simulink model "gm_dsp_proj_v3_2024_n"  (R2025b)
settings: Solver=FixedStepDiscrete  StartTime=0.0  StopTime=1e-4  FixedStep=1.66666666666667e-08  RelTol=1e-3
undefined symbols (not defined in the file or in its folder): b_1, b_2, b_3, dspblkCoreblockFVToolHelper, gcbh
libraries: hdlsllib x11, simulink x4
settings Model: Creator=UTSAB KARAN  LastModifiedBy=souma
settings SolverCC: AutoInsertRateTranBlk=on
settings OptimizationCC: BlockReduction=off  ConditionallyExecuteInputs=off
settings DebuggingCC: InheritedTsInSrcMsg=none  SingleTaskRateTransMsg=error

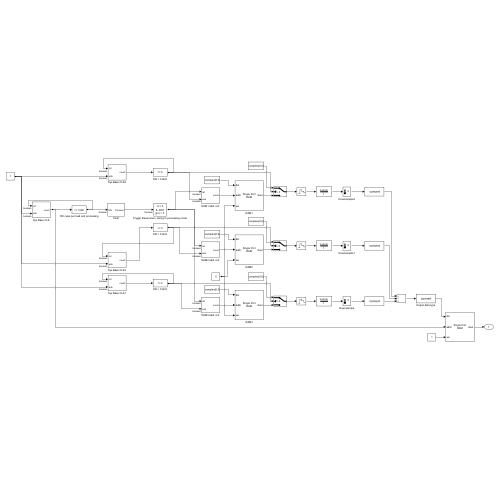
[thumbnail: Simulink's stored preview of the top-level diagram]
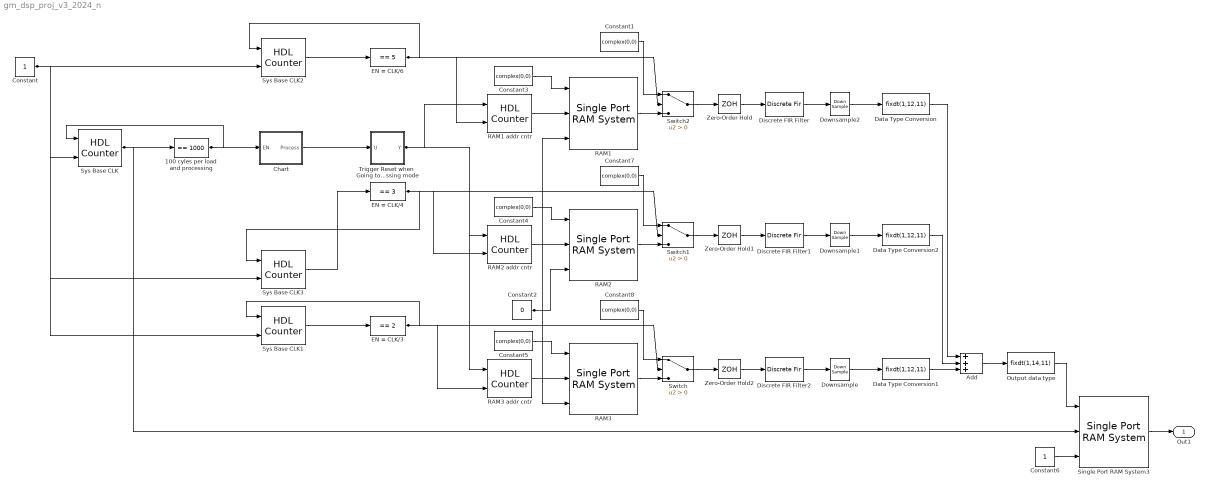
== system gm_dsp_proj_v3_2024_n ==
  100 cyles per load and processing : simulink/Logic and Bit Operations/Compare To Constant  relop===  const=1000  OutDataTypeStr=boolean
  Add : Sum  Inputs=+++  OutDataTypeStr=fixdt(1, 16, 11)
  Chart : Subsystem
  Constant : Constant  OutDataTypeStr=boolean
  Constant1 : Constant  Value=complex(0,0)  VectorParams1D=off  OutDataTypeStr=fixdt(1,8,6)  SampleTime=-1  LockScale=on
  Constant2 : Constant  Value=0  OutDataTypeStr=boolean
  Constant3 : Constant  Value=complex(0,0)  OutDataTypeStr=fixdt(1,8,6)
  Constant4 : Constant  Value=complex(0,0)  OutDataTypeStr=fixdt(1,10,8)
  Constant5 : Constant  Value=complex(0,0)  OutDataTypeStr=fixdt(1,12,10)
  Constant6 : Constant  OutDataTypeStr=boolean
  Constant7 : Constant  Value=complex(0,0)  VectorParams1D=off  OutDataTypeStr=fixdt(1,10,8)  SampleTime=-1  LockScale=on
  Constant8 : Constant  Value=complex(0,0)  VectorParams1D=off  OutDataTypeStr=fixdt(1,12,10)  SampleTime=-1  LockScale=on
  Data Type Conversion : DataTypeConversion  OutDataTypeStr=fixdt(1,12,11)  RndMeth=Floor
  Data Type Conversion1 : DataTypeConversion  OutDataTypeStr=fixdt(1,12,11)  RndMeth=Floor
  Data Type Conversion2 : DataTypeConversion  OutDataTypeStr=fixdt(1,12,11)  RndMeth=Floor
  Discrete FIR Filter : DiscreteFir  LoadFcn=dspblkCoreblockFVToolHelper(gcbh,'load');  FilterStructure=Direct form symmetric  Coefficients=b_1  CoefDataTypeStr=fixdt(1,25,24)  OutDataTypeStr=fixdt(1, 64, 30)
      settings: CopyFcn=dspblkCoreblockFVToolHelper(gcbh,'copy');  DeleteFcn=dspblkCoreblockFVToolHelper(gcbh,'close');  ModelCloseFcn=dspblkCoreblockFVToolHelper(gcbh,'close');  PreSaveFcn=dspblkCoreblockFVToolHelper(gcbh,'presave');  PostSaveFcn=dspblkCoreblockFVToolHelper(gcbh,'postsave');  CloseFcn=dspblkCoreblockFVToolHelper(gcbh,'close');
  Discrete FIR Filter1 : DiscreteFir  LoadFcn=dspblkCoreblockFVToolHelper(gcbh,'load');  FilterStructure=Direct form symmetric  Coefficients=b_2  CoefDataTypeStr=fixdt(1,25,24)  OutDataTypeStr=fixdt(1, 64, 32)
      settings: CopyFcn=dspblkCoreblockFVToolHelper(gcbh,'copy');  DeleteFcn=dspblkCoreblockFVToolHelper(gcbh,'close');  ModelCloseFcn=dspblkCoreblockFVToolHelper(gcbh,'close');  PreSaveFcn=dspblkCoreblockFVToolHelper(gcbh,'presave');  PostSaveFcn=dspblkCoreblockFVToolHelper(gcbh,'postsave');  CloseFcn=dspblkCoreblockFVToolHelper(gcbh,'close');
  Discrete FIR Filter2 : DiscreteFir  LoadFcn=dspblkCoreblockFVToolHelper(gcbh,'load');  FilterStructure=Direct form symmetric  Coefficients=b_3  CoefDataTypeStr=fixdt(1,25,24)  OutDataTypeStr=fixdt(1, 64, 34)
      settings: CopyFcn=dspblkCoreblockFVToolHelper(gcbh,'copy');  DeleteFcn=dspblkCoreblockFVToolHelper(gcbh,'close');  ModelCloseFcn=dspblkCoreblockFVToolHelper(gcbh,'close');  PreSaveFcn=dspblkCoreblockFVToolHelper(gcbh,'presave');  PostSaveFcn=dspblkCoreblockFVToolHelper(gcbh,'postsave');  CloseFcn=dspblkCoreblockFVToolHelper(gcbh,'close');
  Downsample : DownSample  N=5  RateOptions=Allow multirate processing
  Downsample1 : DownSample  N=5  RateOptions=Allow multirate processing
  Downsample2 : DownSample  N=5  RateOptions=Allow multirate processing
  EN = CLK/3 : simulink/Logic and Bit Operations/Compare To Constant  relop===  const=2  OutDataTypeStr=boolean
  EN = CLK/4 : simulink/Logic and Bit Operations/Compare To Constant  relop===  const=3  OutDataTypeStr=boolean
  EN = CLK/6 : simulink/Logic and Bit Operations/Compare To Constant  relop===  const=5  OutDataTypeStr=boolean
  Output data type : DataTypeConversion  OutDataTypeStr=fixdt(1,14,11)  SaturateOnIntegerOverflow=off  RndMeth=Floor  LockScale=on
  RAM1 : hdlsllib/HDL RAMs/Single Port RAM System  RAMType=Single port  AsyncRead=off  WriteOutputValue=New data  RAMInitialValue=ram1_init_data  allowBusInputs=off  WritesHaveOutput=on  NumReads=0  NumWrites=1  SimulateUsing=Code generation  ModelRAMDelay=on  VectorAccess=Parallel
  RAM1 addr cntr : hdlsllib/Sources/HDL Counter  CountType=Count limited  CountInit=0  CountStep=1  CountMax=3000  CountFromType=Initial value  CountFrom=0  CountResetPort=on  CountLoadPort=off  CountEnbPort=on  CountDirPort=off  CountHitOutputPort=off  CountDataType=Unsigned  CountWordLen=12  CountFracLen=0  CountSampTime=1
  RAM2 : hdlsllib/HDL RAMs/Single Port RAM System  RAMType=Single port  AsyncRead=off  WriteOutputValue=New data  RAMInitialValue=ram2_init_data  allowBusInputs=off  WritesHaveOutput=on  NumReads=0  NumWrites=1  SimulateUsing=Code generation  ModelRAMDelay=on  VectorAccess=Parallel
  RAM2 addr cntr : hdlsllib/Sources/HDL Counter  CountType=Count limited  CountInit=0  CountStep=1  CountMax=3000  CountFromType=Initial value  CountFrom=0  CountResetPort=on  CountLoadPort=off  CountEnbPort=on  CountDirPort=off  CountHitOutputPort=off  CountDataType=Unsigned  CountWordLen=12  CountFracLen=0  CountSampTime=1
  RAM3 : hdlsllib/HDL RAMs/Single Port RAM System  RAMType=Single port  AsyncRead=off  WriteOutputValue=New data  RAMInitialValue=ram3_init_data  allowBusInputs=off  WritesHaveOutput=on  NumReads=0  NumWrites=1  SimulateUsing=Code generation  ModelRAMDelay=on  VectorAccess=Parallel
  RAM3 addr cntr : hdlsllib/Sources/HDL Counter  CountType=Count limited  CountInit=0  CountStep=1  CountMax=3000  CountFromType=Initial value  CountFrom=0  CountResetPort=on  CountLoadPort=off  CountEnbPort=on  CountDirPort=off  CountHitOutputPort=off  CountDataType=Unsigned  CountWordLen=12  CountFracLen=0  CountSampTime=1
  Single Port RAM System3 : hdlsllib/HDL RAMs/Single Port RAM System  RAMType=Single port  AsyncRead=off  WriteOutputValue=New data  RAMInitialValue=0  allowBusInputs=off  WritesHaveOutput=on  NumReads=0  NumWrites=1  SimulateUsing=Code generation  ModelRAMDelay=on  VectorAccess=Parallel
  Switch : Switch  Criteria=u2 > Threshold  OutDataTypeStr=fixdt(1, 12, 10)  SaturateOnIntegerOverflow=off  InputSameDT=off
  Switch1 : Switch  Criteria=u2 > Threshold  OutDataTypeStr=fixdt(1, 10, 8)  SaturateOnIntegerOverflow=off  InputSameDT=off
  Switch2 : Switch  Criteria=u2 > Threshold  OutDataTypeStr=fixdt(1, 8, 6)  SaturateOnIntegerOverflow=off  InputSameDT=off
  Sys Base CLK : hdlsllib/Sources/HDL Counter  CountType=Count limited  CountInit=0  CountStep=1  CountMax=1000  CountFromType=Initial value  CountFrom=0  CountResetPort=on  CountLoadPort=off  CountEnbPort=on  CountDirPort=off  CountHitOutputPort=off  CountDataType=Unsigned  CountWordLen=12  CountFracLen=0  CountSampTime=1
  Sys Base CLK1 : hdlsllib/Sources/HDL Counter  CountType=Count limited  CountInit=0  CountStep=1  CountMax=2  CountFromType=Initial value  CountFrom=0  CountResetPort=on  CountLoadPort=off  CountEnbPort=on  CountDirPort=off  CountHitOutputPort=off  CountDataType=Unsigned  CountWordLen=12  CountFracLen=0  CountSampTime=1
  Sys Base CLK2 : hdlsllib/Sources/HDL Counter  CountType=Count limited  CountInit=0  CountStep=1  CountMax=5  CountFromType=Initial value  CountFrom=0  CountResetPort=on  CountLoadPort=off  CountEnbPort=on  CountDirPort=off  CountHitOutputPort=off  CountDataType=Unsigned  CountWordLen=12  CountFracLen=0  CountSampTime=1
  Sys Base CLK3 : hdlsllib/Sources/HDL Counter  CountType=Count limited  CountInit=0  CountStep=1  CountMax=3  CountFromType=Initial value  CountFrom=0  CountResetPort=on  CountLoadPort=off  CountEnbPort=on  CountDirPort=off  CountHitOutputPort=off  CountDataType=Unsigned  CountWordLen=12  CountFracLen=0  CountSampTime=1
  Trigger Reset when  Going to processing mode : Subsystem  mask(Detect Rise Positive){vinit=double(0), InputProcessing=Elements as channels (sample based), OutDataTypeStr=boolean}
      mask prompts: vinit "Simulink:masks:InitialCondition_MP"; InputProcessing "Simulink:masks:InputProcessing_MP"; OutDataTypeStr "Simulink:masks:OutputDataType_MP"
      mask help: Simulink:masks:DetectRisePositive_MD
      mask init:
      | InputProcessing = 'Elements as channels (sample based)';
      | OutDataTypeStr = 'boolean';
      | vinit = double(0);
      mask TypeOptions InputProcessing: Simulink:masks:ColumnsAsChannelsFrameBased | Simulink:masks:ElementsAsChannelsSampleBased
      mask TypeOptions OutDataTypeStr: Simulink:masks:uint8 | Simulink:masks:boolean
      mask Display: fprintf('U > 0\n&  NOT\nU/z > 0')
  Zero-Order Hold : ZeroOrderHold  SampleTime=1/60e6
  Zero-Order Hold1 : ZeroOrderHold  SampleTime=1/60e6
  Zero-Order Hold2 : ZeroOrderHold  SampleTime=1/60e6
  Out1 : Outport  SampleTime=8.33333333333333e-08
  wires:
  Constant/1 -> Sys Base CLK3/2, Sys Base CLK1/2, Sys Base CLK2/2, Sys Base CLK/2
  100 cyles per load and processing/1 -> Sys Base CLK/1, Chart/1(EN)
  Sys Base CLK/1 -> 100 cyles per load and processing/1, Single Port RAM System3/2
  Sys Base CLK2/1 -> EN = CLK/6/1
  Sys Base CLK1/1 -> EN = CLK/3/1
  Sys Base CLK3/1 -> EN = CLK/4/1
  Switch2/1 -> Zero-Order Hold/1
  Chart/1(Process) -> Trigger Reset when  Going to processing mode/1(U)
  Constant7/1 -> Switch1/1
  EN = CLK/6/1 -> Sys Base CLK2/1, Switch2/2, RAM1 addr cntr/2
  Trigger Reset when  Going to processing mode/1(Y) -> RAM1 addr cntr/1, RAM3 addr cntr/1, RAM2 addr cntr/1
  EN = CLK/4/1 -> Sys Base CLK3/1, Switch1/2, RAM2 addr cntr/2
  RAM3/1 -> Switch/3
  Constant8/1 -> Switch/1
  RAM3 addr cntr/1 -> RAM3/2
  EN = CLK/3/1 -> Sys Base CLK1/1, Switch/2, RAM3 addr cntr/2
  Constant3/1 -> RAM1/1
  RAM1 addr cntr/1 -> RAM1/2
  Constant4/1 -> RAM2/1
  Output data type/1 -> Single Port RAM System3/1
  RAM2 addr cntr/1 -> RAM2/2
  Downsample2/1 -> Data Type Conversion/1
  Constant2/1 -> RAM1/3, RAM3/3, RAM2/3
  Discrete FIR Filter2/1 -> Downsample/1
  Constant5/1 -> RAM3/1
  Constant1/1 -> Switch2/1
  RAM1/1 -> Switch2/3
  RAM2/1 -> Switch1/3
  Data Type Conversion1/1 -> Add/3
  Switch1/1 -> Zero-Order Hold1/1
  Switch/1 -> Zero-Order Hold2/1
  Zero-Order Hold/1 -> Discrete FIR Filter/1
  Zero-Order Hold1/1 -> Discrete FIR Filter1/1
  Zero-Order Hold2/1 -> Discrete FIR Filter2/1
  Discrete FIR Filter/1 -> Downsample2/1
  Discrete FIR Filter1/1 -> Downsample1/1
  Downsample1/1 -> Data Type Conversion2/1
  Downsample/1 -> Data Type Conversion1/1
  Data Type Conversion/1 -> Add/1
  Data Type Conversion2/1 -> Add/2
  Single Port RAM System3/1 -> Out1/1
  Add/1 -> Output data type/1
  Constant6/1 -> Single Port RAM System3/3

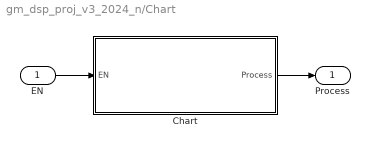
== system gm_dsp_proj_v3_2024_n/Chart ==
  EN : Inport  OutDataTypeStr=boolean  PortDimensions=1  SampleTime=1.66666666666667e-08
  Chart : Stateflow chart  TreatAsAtomicUnit=on
  Process : Outport  SampleTime=1.66666666666667e-08
  wires:
  EN/1 -> Chart/1(EN)
  Chart/1(Process) -> Process/1

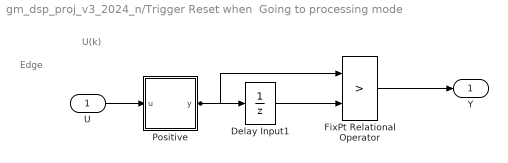
== system gm_dsp_proj_v3_2024_n/Trigger Reset when  Going to processing mode ==
  note: Edge
  note: U(k)
  U : Inport  OutDataTypeStr=boolean  SampleTime=1.66666666666667e-08
  Delay Input1 : UnitDelay  Description=Store in Global RAM  DisableCoverage=on  InitialCondition=vinit  SampleTime=-1  HasFrameUpgradeWarning=on
  FixPt Relational Operator : RelationalOperator  Operator=>  OutDataTypeStr=boolean  ZeroCross=off  InputSameDT=off
  Positive : Subsystem  mask(Compare To Zero){relop=>, OutDataTypeStr=boolean, ZeroCross=off}
      mask prompts: relop "Simulink:masks:Operator_MP"; OutDataTypeStr "Simulink:masks:OutputDataType_MP"; ZeroCross "Simulink:masks:EnableZerocrossingDetection_MP"
      mask help: Simulink:masks:CompareToZero_MD
      mask init:
      | OutDataTypeStr = 'boolean';
      | ZeroCross = 'off';
      | blkName = 'dsp_proj_v3_2024_n/Trigger Reset when \nGoing to processing\nmode/Positive';
      | relop = '>';
      | setValue = 'boolean';
      mask TypeOptions relop: == | ~= | < | <= | >= | >
      mask TypeOptions OutDataTypeStr: Simulink:masks:uint8 | Simulink:masks:boolean
      mask Callback ZeroCross: sl('zeroCrossEnable', gcbh);
      mask Display: disp([relop,' 0'])
  Y : Outport  SampleTime=1.66666666666667e-08  InitialOutput=0
  wires:
  Delay Input1/1 -> FixPt Relational Operator/2
  U/1 -> Positive/1(u)
  FixPt Relational Operator/1 -> Y/1
  Positive/1(y) -> FixPt Relational Operator/1, Delay Input1/1

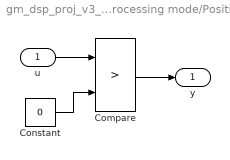
== system gm_dsp_proj_v3_2024_n/Trigger Reset when  Going to processing mode/Positive ==
  u : Inport  OutDataTypeStr=boolean  SampleTime=1.66666666666667e-08
  Compare : RelationalOperator  Operator=>  OutDataTypeStr=boolean  ZeroCross=off
  Constant : Constant  DisableCoverage=on  Value=0  OutDataTypeStr=boolean  SampleTime=-1  PreserveConstantTs=on
  y : Outport  SampleTime=1.66666666666667e-08
  wires:
  u/1 -> Compare/1
  Constant/1 -> Compare/2
  Compare/1 -> y/1

== stateflow chart gm_dsp_proj_v3_2024_n/Chart/Chart ==
  settings: stateMachineType=MOORE_MACHINE  executeAtInitialization=1
  state Processing
    Process = true
  state Data_Loading
    Process = false
  Data_Loading -> Processing : [ EN==1]
  (default) -> Data_Loading
  data: Process output; EN input
